simulink model "task_5"  (R2024a)
settings: Solver=VariableStepAuto  StartTime=0.0  StopTime=25  MaxStep=0.001  RelTol=1e-3
undefined symbols (not defined in the file): ki, kp
settings Model: Creator=kit  LastModifiedBy=sizgr

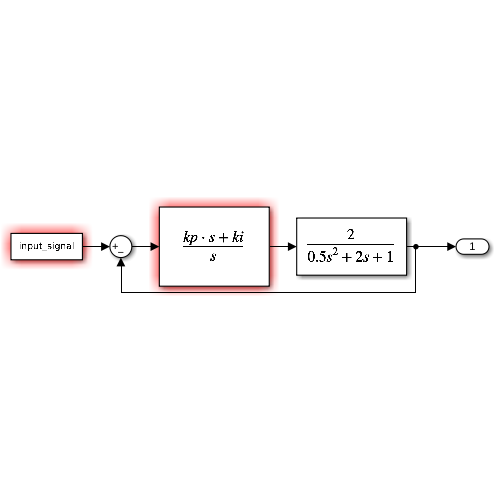
[thumbnail: Simulink's stored preview of the top-level diagram]
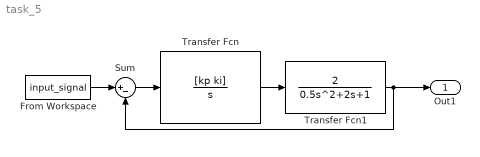
== system task_5 ==
  From Workspace : FromWorkspace  VariableName=input_signal
  Sum : Sum  Inputs=|+-
  Transfer Fcn : TransferFcn  Numerator=[kp ki]  Denominator=[1 0]
  Transfer Fcn1 : TransferFcn  Numerator=[2]  Denominator=[0.5 2 1]
  Out1 : Outport
  wires:
  Sum/1 -> Transfer Fcn/1
  Transfer Fcn/1 -> Transfer Fcn1/1
  Transfer Fcn1/1 -> Sum/2, Out1/1
  From Workspace/1 -> Sum/1
